simulink model "s7_template"  (R2019a)
settings: Solver=ode4  StartTime=0.0  StopTime=inf  FixedStep=P_sim_dt  RelTol=1e-3
InitFcn:
  | s6_data;
values from neighbouring files (symbols this model uses):
  P_sim_dt = 2e-3    (= 0.002)    [s6_data.m]
  psi = p.psi + ((t.a * t.xe.^2) / 2) - (t.a/2) * (t.xe - x).^2    [mbc_clothoid_get_points.m]    (also in s6_data.m = -1.57079632679)
  s1 = p.s1 + integral(fun_cos, 0, xe)    [mbc_clothoid_create.m]
  s2 = p.s2 + integral(fun_sin, 0, xe)    [mbc_clothoid_create.m]
undefined symbols (not defined in the file or in its folder): P_p_Bf, P_p_Br, P_p_Cf, P_p_Cr, P_p_delta_max, P_p_delta_min, P_p_delta_Tt, P_p_Df, P_p_Dr, P_p_frontaxle_1, P_p_J, P_p_k, P_p_l, P_p_m, P_p_output_Tt, P_p_psi0, P_p_psistd, P_p_rearaxle_1, P_p_s10, P_p_s20, P_p_sstd, P_p_T, P_p_un_max, P_p_un_min, P_p_uTt, P_p_v_min, P_p_xvec0
libraries: mad_lib_template x1, realtime_pacer_lib x1
settings Model: Creator=hmekiedj  LastModifiedBy=ftraenkle
settings DataIOCC: ReturnWorkspaceOutputs=off
settings DebuggingCC: ArithmeticOperatorsInVariantConditions=warning
settings SFSimCC: SimUseLocalCustomCode=off
settings RTWCC: RTWUseLocalCustomCode=off

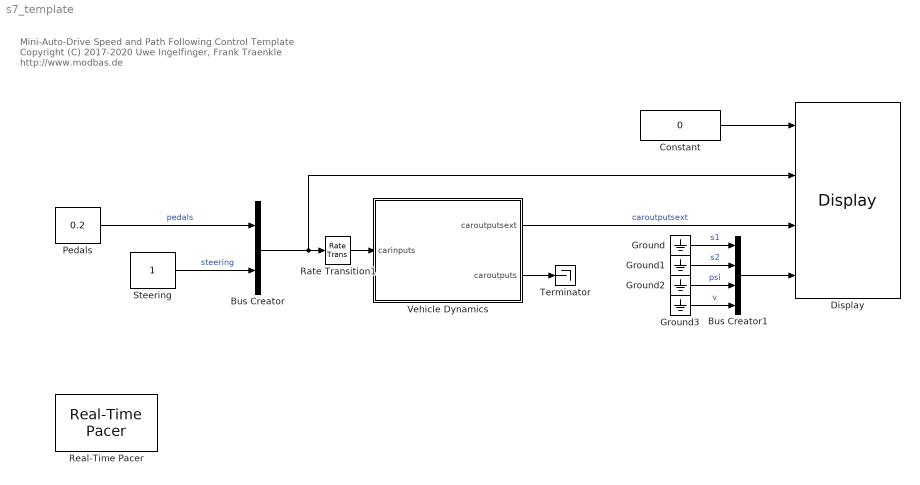
== system s7_template ==
  note: Mini-Auto-Drive
      | Speed and Path Following Control Template
      | Copyright (C) 2017-2020 Uwe Ingelfinger,  Frank Traenkle
      | http://www.modbas.de
  Bus Creator : BusCreator  Inputs=2
  Bus Creator1 : BusCreator  Inputs=4
  Constant : Constant  Value=0
  Display : mad_lib_template/Display  SystemSampleTime=-1
  Ground{,1..3} (4 alike) : Ground
  Pedals : Constant  Value=0.2  SampleTime=-1
  Rate Transition1 : RateTransition
  Real-Time Pacer : realtime_pacer_lib/Real-Time Pacer  simTimePerRealTime=1
  Steering : Constant  SampleTime=-1
  Terminator : Terminator
  Vehicle Dynamics : Subsystem  mask{P_mask_vec0=P_p_xvec0}
      mask prompts: P_mask_vec0 "Initial vale"
  wires:
  Bus Creator/1 -> Display/2, Rate Transition1/1
  Bus Creator1/1 -> Display/4
  Ground/1 -> Bus Creator1/1  "s1"
  Ground1/1 -> Bus Creator1/2  "s2"
  Ground2/1 -> Bus Creator1/3  "psi"
  Ground3/1 -> Bus Creator1/4  "v"
  Vehicle Dynamics/1(caroutputsext) -> Display/3  "caroutputsext"
  Vehicle Dynamics/2(caroutputs) -> Terminator/1
  Pedals/1 -> Bus Creator/1  "pedals"
  Steering/1 -> Bus Creator/2  "steering"
  Rate Transition1/1 -> Vehicle Dynamics/1(carinputs)
  Constant/1 -> Display/1

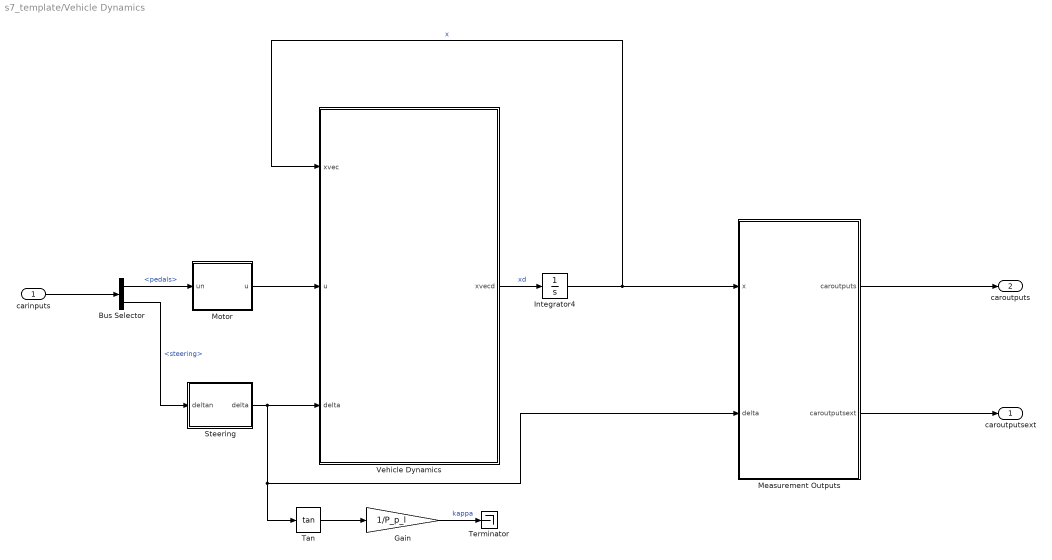
== system s7_template/Vehicle Dynamics ==
  carinputs : Inport
  Bus Selector : BusSelector  OutputSignals=pedals,steering
  Gain : Gain  Gain=1/P_p_l
  Integrator4 : Integrator  InitialCondition=P_mask_vec0
  Measurement Outputs : Subsystem
  Motor : Subsystem
  "Steering " : Subsystem
  Tan : Trigonometry  Operator=tan
  Terminator : Terminator
  Vehicle Dynamics : MATLAB Function  TreatAsAtomicUnit=on
  caroutputsext : Outport
  caroutputs : Outport  Port=2
  wires:
  carinputs/1 -> Bus Selector/1
  Motor/1(u) -> Vehicle Dynamics/2(u)
  "Steering "/1(delta) -> Tan/1, Measurement Outputs/2(delta), Vehicle Dynamics/3(delta)
  Vehicle Dynamics/1(xvecd) -> Integrator4/1  "xd"
  Integrator4/1 -> Vehicle Dynamics/1(xvec), Measurement Outputs/1(x)  "x"
  Bus Selector/1 -> Motor/1(un)  "<pedals>"
  Bus Selector/2 -> "Steering "/1(deltan)  "<steering>"
  Measurement Outputs/1(caroutputs) -> caroutputs/1
  Measurement Outputs/2(caroutputsext) -> caroutputsext/1
  Tan/1 -> Gain/1
  Gain/1 -> Terminator/1  "kappa"

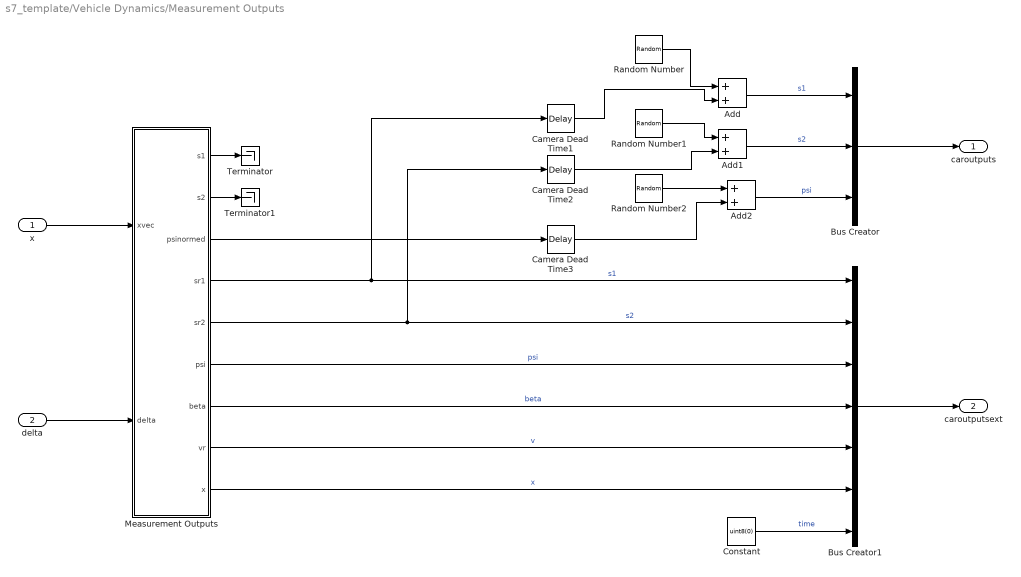
== system s7_template/Vehicle Dynamics/Measurement Outputs ==
  x : Inport
  delta : Inport  Port=2
  Add : Sum
  Add1 : Sum
  Add2 : Sum
  Bus Creator : BusCreator  Inputs=s1,s2,psi  OutDataTypeStr=Bus: CAROUTPUTS  NonVirtualBus=on
  Bus Creator1 : BusCreator  Inputs=7  OutDataTypeStr=Bus: CAROUTPUTSEXT  NonVirtualBus=on
  Camera Dead Time1 : TransportDelay  DelayTime=P_p_output_Tt  InitialOutput=P_p_s10  FixedBuffer=on
  Camera Dead Time2 : TransportDelay  DelayTime=P_p_output_Tt  InitialOutput=P_p_s20  FixedBuffer=on
  Camera Dead Time3 : TransportDelay  DelayTime=P_p_output_Tt  InitialOutput=P_p_psi0  FixedBuffer=on
  Constant : Constant  Value=uint8(0)
  Measurement Outputs : MATLAB Function  TreatAsAtomicUnit=on
  Random Number : RandomNumber  Variance=P_p_sstd^2  SampleTime=P_sim_dt
  Random Number1 : RandomNumber  Variance=P_p_sstd^2  Seed=1  SampleTime=P_sim_dt
  Random Number2 : RandomNumber  Variance=P_p_psistd^2  Seed=2  SampleTime=P_sim_dt
  Terminator : Terminator
  Terminator1 : Terminator
  caroutputs : Outport
  caroutputsext : Outport  Port=2
  wires:
  Measurement Outputs/4(sr1) -> Camera Dead Time1/1, Bus Creator1/1  "s1"
  Measurement Outputs/7(beta) -> Bus Creator1/4  "beta"
  Measurement Outputs/8(vr) -> Bus Creator1/5  "v"
  Measurement Outputs/9(x) -> Bus Creator1/6  "x"
  Measurement Outputs/5(sr2) -> Bus Creator1/2, Camera Dead Time2/1  "s2"
  Bus Creator/1 -> caroutputs/1
  Bus Creator1/1 -> caroutputsext/1
  x/1 -> Measurement Outputs/1(xvec)
  Camera Dead Time1/1 -> Add/2
  Random Number/1 -> Add/1
  Add/1 -> Bus Creator/1  "s1"
  Random Number1/1 -> Add1/1
  Camera Dead Time2/1 -> Add1/2
  Add1/1 -> Bus Creator/2  "s2"
  Camera Dead Time3/1 -> Add2/2
  Random Number2/1 -> Add2/1
  Add2/1 -> Bus Creator/3  "psi"
  delta/1 -> Measurement Outputs/2(delta)
  Measurement Outputs/3(psinormed) -> Camera Dead Time3/1
  Measurement Outputs/6(psi) -> Bus Creator1/3  "psi"
  Constant/1 -> Bus Creator1/7  "time"
  Measurement Outputs/1(s1) -> Terminator/1
  Measurement Outputs/2(s2) -> Terminator1/1

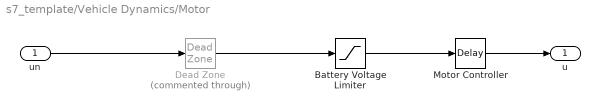
== system s7_template/Vehicle Dynamics/Motor ==
  un : Inport
  Battery Voltage Limiter : Saturate  UpperLimit=P_p_un_max  LowerLimit=P_p_un_min
  Dead Zone : DeadZone  Commented=through  LowerValue=P_p_un_friction_neg  UpperValue=P_p_un_friction_pos  SaturateOnIntegerOverflow=on
  Motor Controller : TransportDelay  DelayTime=P_p_uTt  FixedBuffer=on
  u : Outport
  wires:
  Battery Voltage Limiter/1 -> Motor Controller/1
  Motor Controller/1 -> u/1
  un/1 -> Dead Zone/1
  Dead Zone/1 -> Battery Voltage Limiter/1

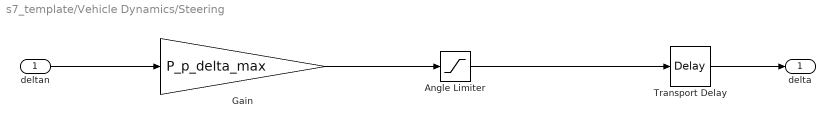
== system s7_template/Vehicle Dynamics/Steering  ==
  deltan : Inport
  Angle Limiter : Saturate  UpperLimit=P_p_delta_max  LowerLimit=P_p_delta_min
  Gain : Gain  Gain=P_p_delta_max
  Transport Delay : TransportDelay  DelayTime=P_p_delta_Tt  FixedBuffer=on
  delta : Outport
  wires:
  deltan/1 -> Gain/1
  Gain/1 -> Angle Limiter/1
  Transport Delay/1 -> delta/1
  Angle Limiter/1 -> Transport Delay/1

== matlab function s7_template/Vehicle Dynamics/Measurement Outputs/Measurement Outputs ==
  data: xvec input; delta input; s1 output; s2 output; psinormed output; sr1 output; sr2 output; psi output; beta output; vr output; x output; P_p_rearaxle_1 parameter; P_p_v_min parameter; P_p_l parameter
function [s1, s2, psinormed, sr1, sr2, psi, beta, vr, x] = outputs(xvec, delta, P_p_rearaxle_1, P_p_v_min, P_p_l)
%#codegen
vc1 = xvec(1);
s1 = xvec(2);
s2 = xvec(3);
psi = xvec(4);
x = xvec(7);

psinormed = mod(psi, 2*pi);
if psinormed > pi
    psinormed = psinormed - 2*pi;
end
beta = 0;
sr1 = s1 - P_p_rearaxle_1 * cos(psi);
sr2 = s2 - P_p_rearaxle_1 * sin(psi);
vr = vc1;
end

== matlab function s7_template/Vehicle Dynamics/Vehicle Dynamics ==
  data: xvec input; u input; xvecd output; delta input; P_p_Br parameter; P_p_Bf parameter; P_p_Cr parameter; P_p_Cf parameter; P_p_Dr parameter; P_p_Df parameter; P_p_rearaxle_1 parameter; P_p_frontaxle_1 parameter; P_p_m parameter; P_p_J parameter; P_p_k parameter; P_p_T parameter; P_p_v_min parameter; P_p_l parameter
function xvecd = dynamics(xvec, u, delta, P_p_Br, P_p_Bf, P_p_Cr, P_p_Cf, P_p_Dr, P_p_Df, ...
    P_p_rearaxle_1, P_p_frontaxle_1, P_p_m, P_p_J, P_p_k, P_p_T, P_p_v_min, P_p_l)
%#codegen

vc1 = xvec(1);
psi = xvec(4);
psid = xvec(5);
vc2 = xvec(6);

if abs(vc1) > P_p_v_min % avoid model singularity at zero speed
    %% bicycle model with Magic Tire
    spsi = sin(psi);
    cpsi = cos(psi);
    sdelta = sin(delta);
    cdelta = cos(delta);
    
    % wheel slip angles
    alphaf = -atan2(vc2 + P_p_frontaxle_1 * psid, vc1) + delta;
    alphar = -atan2(vc2 - P_p_rearaxle_1 * psid, vc1);
    % wheel forces
    Ff = P_p_Df * sin(P_p_Cf * atan(P_p_Bf * alphaf));
    Fr = P_p_Dr * sin(P_p_Cr * atan(P_p_Br * alphar));    
    % logitudinal dynamics (momentum balance)
    vc1d = (-Ff * sdelta + P_p_m * vc2 * psid) / P_p_m ...
            - vc1/P_p_T + P_p_k/P_p_T * u;
    % kinematics
    s1d = vc1 * cpsi - vc2 * spsi;
    s2d = vc1 * spsi + vc2 * cpsi;
    % rotational dynamics (moment of momentum balance)
    psidd = (Ff * P_p_frontaxle_1 * cdelta - Fr * P_p_rearaxle_1) / P_p_J;
    % lateral dynamics (momentum balance)
    vc2d = (Ff * cdelta + Fr - P_p_m * vc1 * psid)/P_p_m;
    % driven arc length of rear axle center
    xd = vc1;
else % near zero speed
    %% longitudinal dynamics of rear axle
    a = P_p_rearaxle_1;
    l = P_p_l;
    spsi = sin(psi);
    cpsi = cos(psi);
    tdelta = tan(delta);
    vc2 = a/l * vc1 * tdelta;
    vc1d = (-vc1 + P_p_k * u) / P_p_T; % -(a^2+P_p_J/P_p-m)/l^2*vc1*tdelta*deltad
    s1d = vc1 * cpsi - vc2 * spsi;
    s2d = vc1 * spsi + vc2 * cpsi;
    psid = vc1 / l * tdelta;
    psidd = 0; % vc1d / l * tdelta + vc1/l * deltad * (1 + tdelta*delta)
    vc2d = 0 ; % a * psidd;
    xd = vc1;
end
    
xvecd = [ vc1d; s1d; s2d; psid; psidd; vc2d; xd ];
end
